simulink model "DEMO_generalDistributionRouting"  (R2015b)
settings: Solver=VariableStepAuto  StartTime=0.0  StopTime=10000  RelTol=1e-3
undefined symbols (not defined in the file or in its folder): des
settings Model: Creator=tsprock3  LastModifiedBy=tsprock3
settings DebuggingCC: UnconnectedOutputMsg=error

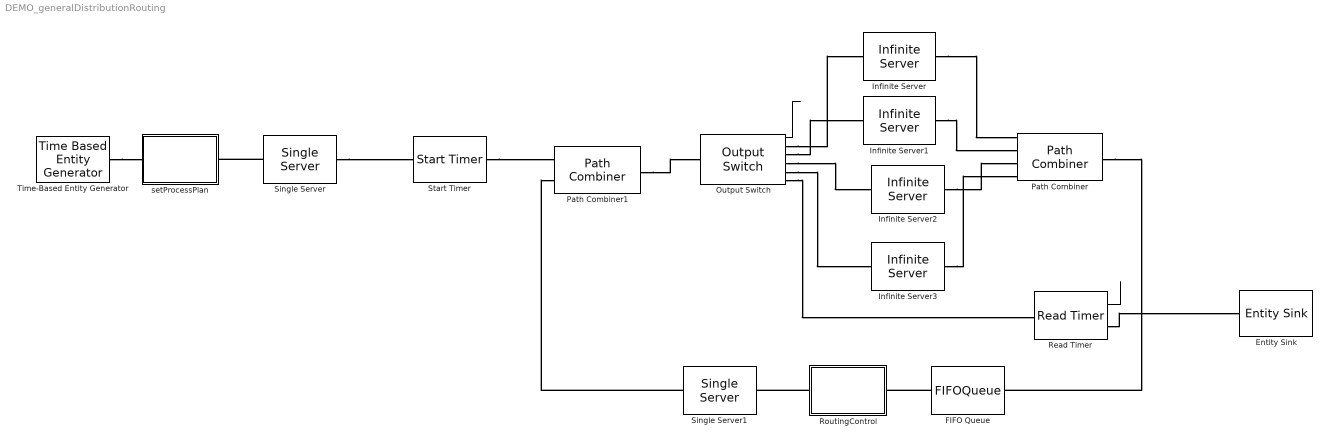
== system DEMO_generalDistributionRouting ==
  Entity Sink : EntitySink
  FIFO Queue : FIFOQueue
  Infinite Server{,1..3} (4 alike) : InfiniteServer
  Output Switch : OutputSwitch  NumberOutputPorts=5  SwitchingCriterion=From attribute  AttributeName=NextProcess  StatLastDeparturePort=on
      settings: OutputPortMap=o3
  Path Combiner : PathCombiner  NumberInputPorts=4
  Path Combiner1 : PathCombiner  NumberInputPorts=2
  Read Timer : ReadTimer  StatTimeElapsed=on
      settings: OutputPortMap=o2
  RoutingControl : Subsystem  LoadFcn=des.afb.attributefunction_support(gcb,'LoadFcn');  StartFcn=des.afb.attributefunction_support(gcb,'StartFcn');  mask(Attribute Function){OutputNamePrefix=out_}
      mask prompts: OutputNamePrefix "Prefix name"
      settings: CopyFcn=des.afb.attributefunction_support(gcb,'CopyFcn');  OpenFcn=des.afb.attributefunction_support(gcb,'OpenFcn');  ErrorFcn=des.afb.error_redirect
      mask Help: slhelp(gcbh)
      mask Display: image(des_iconLoad('attribFunction.jpg'),'center');
  Single Server : SingleServer  ServiceTime=0
  Single Server1 : SingleServer  ServiceTime=0
  Start Timer : StartTimer
  Time-Based Entity Generator : TimeBasedEntityGenerator
  setProcessPlan : Subsystem  LoadFcn=des.afb.attributefunction_support(gcb,'LoadFcn');  StartFcn=des.afb.attributefunction_support(gcb,'StartFcn');  mask(Attribute Function){OutputNamePrefix=out_}
      mask prompts: OutputNamePrefix "Prefix name"
      settings: CopyFcn=des.afb.attributefunction_support(gcb,'CopyFcn');  OpenFcn=des.afb.attributefunction_support(gcb,'OpenFcn');  ErrorFcn=des.afb.error_redirect
      mask Help: slhelp(gcbh)
      mask Display: image(des_iconLoad('attribFunction.jpg'),'center');
  wires:
  Output Switch/1 -> ?
  Read Timer/1 -> ?
  connections:
  Single Server/LConn1 -- setProcessPlan/RConn1
  Path Combiner1/RConn1 -- Output Switch/LConn1
  RoutingControl/RConn1 -- Single Server1/LConn1
  FIFO Queue/RConn1 -- RoutingControl/LConn1
  Time-Based Entity Generator/RConn1 -- setProcessPlan/LConn1
  Path Combiner/RConn1 -- FIFO Queue/LConn1
  Single Server1/RConn1 -- Path Combiner1/LConn2
  Output Switch/RConn1 -- Infinite Server/LConn1
  Output Switch/RConn2 -- Infinite Server1/LConn1
  Output Switch/RConn3 -- Infinite Server2/LConn1
  Output Switch/RConn4 -- Infinite Server3/LConn1
  Infinite Server/RConn1 -- Path Combiner/LConn1
  Infinite Server1/RConn1 -- Path Combiner/LConn2
  Infinite Server2/RConn1 -- Path Combiner/LConn3
  Infinite Server3/RConn1 -- Path Combiner/LConn4
  Single Server/RConn1 -- Start Timer/LConn1
  Start Timer/RConn1 -- Path Combiner1/LConn1
  Output Switch/RConn5 -- Read Timer/LConn1
  Read Timer/RConn1 -- Entity Sink/LConn1

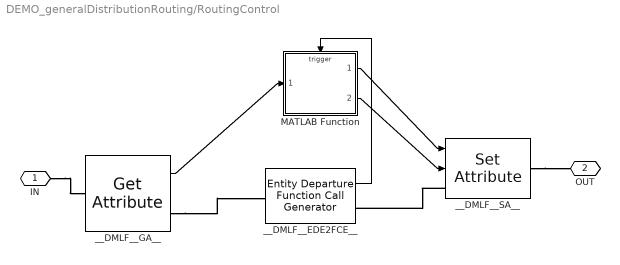
== system DEMO_generalDistributionRouting/RoutingControl ==
  MATLAB Function : MATLAB Function  TreatAsAtomicUnit=on
  __DMLF__EDE2FCE__ : EntityDepartureFunctionCallGenerator  TimingFunctionCallF1=Before entity departure  IsInsideAFB=on
  __DMLF__GA__ : GetAttribute  AttributeName=ProcessPlan  AttributeSendTiming=Before entity departure  EvaluatedDefaultAttributeValue={ []}  IsInsideAFB=on
      settings: OutputPortMap=o1
  __DMLF__SA__ : SetAttribute  AttributeName=ProcessPlan|NextProcess  AttributeFrom=Signal port|Signal port  AttributeValue=1|1  AttributeTreatAsVector=1|1  EvaluatedAttributeValue={ [];[]}  IsInsideAFB=on
      settings: InputPortMap=u0,u1
  IN : PMIOPort  Port=1  Side=Left
  OUT : PMIOPort  Port=2  Side=Right
  wires:
  __DMLF__EDE2FCE__/1 -> MATLAB Function/Trigger
  __DMLF__GA__/1 -> MATLAB Function/1(ProcessPlan)
  MATLAB Function/1(out_ProcessPlan) -> __DMLF__SA__/1
  MATLAB Function/2(out_NextProcess) -> __DMLF__SA__/2
  connections:
  __DMLF__SA__/LConn1 -- __DMLF__EDE2FCE__/RConn1
  __DMLF__GA__/RConn1 -- __DMLF__EDE2FCE__/LConn1
  IN/RConn1 -- __DMLF__GA__/LConn1
  __DMLF__SA__/RConn1 -- OUT/RConn1

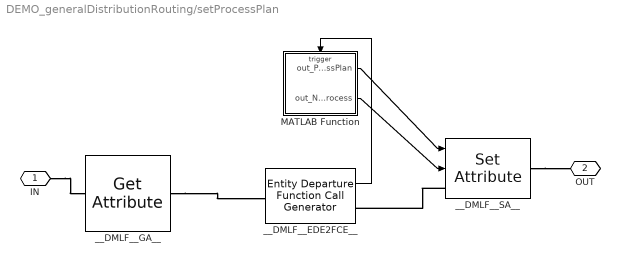
== system DEMO_generalDistributionRouting/setProcessPlan ==
  MATLAB Function : MATLAB Function  TreatAsAtomicUnit=on
  __DMLF__EDE2FCE__ : EntityDepartureFunctionCallGenerator  TimingFunctionCallF1=Before entity departure  IsInsideAFB=on
  __DMLF__GA__ : GetAttribute  EvaluatedDefaultAttributeValue={ }  IsInsideAFB=on
  __DMLF__SA__ : SetAttribute  AttributeName=ProcessPlan|NextProcess  AttributeFrom=Signal port|Signal port  AttributeValue=1|1  AttributeTreatAsVector=1|1  EvaluatedAttributeValue={ [];[]}  IsInsideAFB=on
      settings: InputPortMap=u0,u1
  IN : PMIOPort  Port=1  Side=Left
  OUT : PMIOPort  Port=2  Side=Right
  wires:
  __DMLF__EDE2FCE__/1 -> MATLAB Function/Trigger
  MATLAB Function/1(out_ProcessPlan) -> __DMLF__SA__/1
  MATLAB Function/2(out_NextProcess) -> __DMLF__SA__/2
  connections:
  __DMLF__SA__/LConn1 -- __DMLF__EDE2FCE__/RConn1
  __DMLF__GA__/RConn1 -- __DMLF__EDE2FCE__/LConn1
  IN/RConn1 -- __DMLF__GA__/LConn1
  __DMLF__SA__/RConn1 -- OUT/RConn1

== matlab function DEMO_generalDistributionRouting/setProcessPlan/MATLAB Function ==
  data: out_ProcessPlan output; out_NextProcess output
  events: trigger input FUNCTION_CALL_EVENT
function [out_ProcessPlan, out_NextProcess] = fcn()
%FCN    Access and modify attributes with MATLAB 


Q = [0.33 0.33 0.34]; %P(Length of Process Plan)
P = [0.25 0.25 0.25 0.25]; %P(Visit Station k)

%Using the coder.extrinsic to hide all of the generateProcessPlan details
%greatly simplifies the hurdles for simulink.
coder.extrinsic('generateProcessPlan');

%Initialize the output variables to the correct dimensions (dimensions
%cannot change during simulink run)
out_ProcessPlan = coder.nullcopy(zeros(length(Q)+1,1)); %must be the length of the longest process plan + 1
out_NextProcess = coder.nullcopy(zeros(1,1));

[ProcessPlan, NextProcess] = generateProcessPlan(length(Q), Q, P);

out_ProcessPlan = ProcessPlan;
out_NextProcess = NextProcess;

== matlab function DEMO_generalDistributionRouting/RoutingControl/MATLAB Function ==
  data: ProcessPlan input; out_ProcessPlan output; out_NextProcess output
  events: trigger input FUNCTION_CALL_EVENT
function [out_ProcessPlan, out_NextProcess] = fcn(ProcessPlan)

if ProcessPlan(1) == 0
    %Covers the initialization of the simulation
    out_NextProcess = 1;
else
    out_NextProcess = ProcessPlan(1);
end

out_ProcessPlan = ProcessPlan([2:end 1]);
    
end
